simulink model "experimental_1026"  (Simulink 7.5)
settings: Solver=ode1  StartTime=0.0  StopTime=Inf  FixedStep=1/12000  RelTol=1e-3
PostLoadFcn:
  | , if any(exist('dsrtsu_mdlpostloadfcn', 'file') == [2, 3, 6]), try dsrtsu_mdlpostloadfcn('Execute', bdroot); catch fprintf('Error in PostLoadFcn (dsrtsu_mdlpostloadfcn) for model "%s":\n %s\n', bdroot, lasterr); end, end,
InitFcn:
  | iC_ini
values from neighbouring files (symbols this model uses):
  Ts = 0.5    [IMC_calculo_limites_thetas.m]    (also in IMC_datta_ini.m; IMC_ini.m = 8.33333333333e-05; JORGE_controlador_LCL_malha_interna.m = 8.33333333333e-05; LCL_PAPM.m = 8.33333333333e-05)
libraries: powerlib x7, rtilib1103 x2, simulink x1, dsextras x1
CloseFcn:
  | rtwprivate ssgensfun ModelCloseRequest experimental_1021
settings Model: DSRTSU_INTERNAL_RTI_VER=390  DSRTSU_INTERNAL_RTI_TYPE=rti1103  Creator=dpbernardon  LastModifiedBy=dpbernardon  BufferReuse=off
settings SolverCC: InsertRTBMode=Always
settings OptimizationCC: BlockReduction=off  OptimizeBlockIOStorage=off  BufferReuse=off  ExpressionFolding=off  LocalBlockOutputs=off
settings HardwareCC: ProdIntDivRoundTo=Zero  ProdEndianess=BigEndian  ProdHWDeviceType=Generic->Custom  TargetIntDivRoundTo=Zero  TargetEndianess=BigEndian  TargetHWDeviceType=Generic->Custom
settings RTWCC: SystemTargetFile=rti1103.tlc  MakeCommand=make_rti  TemplateMakefile=rti1103.tmf  Description=dSPACE DS1103 Hardware Platform  ProcessScript=rti1103_make_rtw_hook
settings STFCustomTargetCC: ParMdlRefBuildCompliant=on  GeneratePreprocessorConditionals=Disable all  SystemTargetFile=rti1103.tlc
settings GRTTargetCC: CompOptLevelCompliant=off  MatFileLogging=off  ExtModeMexFile=noextcomm
settings CustomProperty: DataType=RTWOptions_EnumType_C__dSPACE RCPHIL 72_matlab_rti1103_tlc_rti1103_1InitialSimState  Value=RUN
settings EnumStrPairs: String=RUN

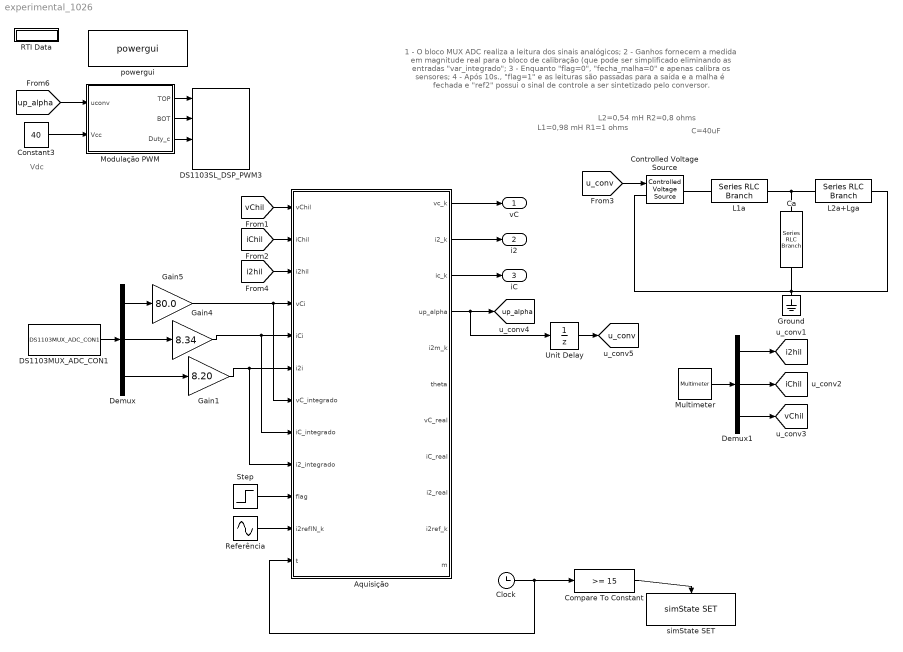
== system experimental_1026 ==
  note: Vdc
  note: 1 - O bloco MUX ADC realiza a leitura dos sinais analógicos;
      | 2 - Ganhos fornecem a medida em magnitude real para o bloco de calibração (que pode ser simplificado  eliminando as entradas "var_integrado";
      | 3 - Enquanto "flag=0", "fecha_malha=0" e apenas calibra os sensores;
      | 4 - Após 10s., "flag=1" e as leituras são passadas para a saída e a malha é fechada e "ref2" possui o sinal de controle a ser sintetizado pelo conversor.
  note: L1=0,98 mH
      | R1=1 ohms
  note: L2=0,54 mH
      | R2=0,8 ohms
  note: C=40uF
  Aquisição : Stateflow chart  TreatAsAtomicUnit=on  SystemSampleTime=Ts
      settings: MinAlgLoopOccurrences=on  RTWSystemCode=Function
  Ca : powerlib/Elements/Series RLC Branch  DialogController=POWERSYS.PowerSysDialog  PhysicalDomain=powersysdomain  SubClassName=unknown  LeftPortType=p1  RightPortType=p1  LConnTagsString=__new0  RConnTagsString=__new0  BranchType=C  Resistance=1  Inductance=1e-3  SetiL0=off  InitialCurrent=0  Capacitance=0.000040  Setx0=off  InitialVoltage=0  Measurements=Branch voltage and current
  Clock : Clock
      settings: Decimation=10
  Compare To Constant : simulink/Logic and Bit Operations/Compare To Constant  SystemSampleTime=-1  relop=>=  const=15  LogicOutDataTypeMode=uint8
  Constant3 : Constant  Value=40  OutDataType=fixdt(1, 16)  OutScaling=2^0
  Controlled Voltage Source : powerlib/Electrical Sources/Controlled Voltage Source  DialogController=POWERSYS.PowerSysDialog  SystemSampleTime=-1  Initialize=on  Source_Type=AC  Amplitude=0  Phase=0  Frequency=0  Measurements=None
  DS1103MUX_ADC_CON1 : rtilib1103/DS1103 MASTER PPC/DS1103MUX_ADC_CON1  SystemSampleTime=-1  ConverterNo=1  ChannelNos=[1 2 3]  TimerAPreTrigger=0  Reserved2=[]  Reserved3=[]  Reserved4=[]  DialogFcn=gui1103mux_adc  UnitName={ 'DS1103MUX_ADC_CON' }  UnitValues={ 1 }  DSProperties=struct('RTI',struct('Version',uint32(1),'BlockType',struct('isSLSource',uint8(1),'isSLSink',uint8(0),'isHWSource',uint8(1),'isHWSink',uint8(0),'isSetup',uint8(0),'isInline',uint8(1),'isNonInline',uint8(0),'isInterrupt',uint8(0),'isChannelwise',uint8(0)),'IOBoardType','DS1103MASTER','UnitType','ADC','Identifier','ADCMUX','DialogType','ML','BlockSet','NONE','SlaveProcessor','NONE'))
  DS1103SL_DSP_PWM3 : rtilib1103/DS1103 SLAVE DSP/DS1103SL_DSP_PWM3  SystemSampleTime=-1  Parameters=[]  TDef=[]  BoardType=[]  PwmMode=[]  Frequency=[]  DeadBand=[]  InitValue=[]  TermMode=[]  TermValue=[]  IntDelay=[]  DialogFcn=[]  Reserved1=[]  Reserved2=[]  Reserved3=[]  Reserved4=[]  Revision=[]  UnitName=[]  UnitValues=[]  DSProperties=struct('RTI',struct('Version',uint32(2),'BlockType',struct('isSLSource',uint8(0),'isSLSink',uint8(1),'isHWSource',uint8(0),'isHWSink',uint8(1),'isSetup',uint8(0),'isInline',uint8(1),'isNonInline',uint8(0),'isInterrupt',uint8(0),'isChannelwise',uint8(0)),'IOBoardType','DS1103SLAVE','UnitType','PWM','Identifier','PWM3','DialogType','ML','BlockSet','NONE','SlaveProcessor','F240'))  RTIBlockInterface=struct('InputPortsActive',[1 1 1 1],'InputPortsWidth',int32([1 1 1 1]),'InputPortsName',{{['Duty cycle a'],['Duty cycle b'],['Duty cycle c'],['PWM Stop']}},'IWork',{{{'',uint32(1)}}},'DialogFcn','rti1103slavepwm3gui','InitLevel',1,'BlockDisplay',{{'','auto'}},'IconTransparency','on','BlockName',struct('Token',{{'DS1103SL_DSP_PWM3'}}))  RTIBlockParameters=struct('PWMFrequency',{{'12000','OFF',[]}},'PWMDeadband',{{'2','OFF',[]}},'PWMPolarityMode',{{[1 1 1 1],'OFF',[]}},'PWMPolarityInvMode',{{[2 2 2 2],'OFF',[]}},'SuspendModeInit',{{[1 1 1],'OFF',[]}},'TTLModeInit',{{[1 1 1],'OFF',[]}},'TTLModeInitNOT',{{[2 2 2],'OFF',[]}},'DutyCycleInitValueCh1',{{'0.5','OFF',[]}},'DutyCycleInitValueCh2',{{'0.5','OFF',[]}},'DutyCycleInitValueCh3',{{'0.5','OFF',[]}},'EnablePWMStop',{{1,'OFF',[]}},'SuspendModeTerm',{{[1 1 1],'OFF',[]}},'TTLModeTerm',{{[1 1 1],'OFF',[]}},'TTLModeTermNOT',{{[2 2 2],'OFF',[]}},'DutyCycleTermValueCh1',{{'0.5','OFF',[]}},'DutyCycleTermValueCh2',{{'0.5','OFF',[]}},'DutyCycleTermValueCh3',{{'0.5','OFF',[]}},'TLCFileName',{{'rti1103pwm3','OFF',[]}})  RTISFcnParameters=struct('PWMFrequency','double','PWMDeadband','double','PWMPolarityMode','double','PWMPolarityInvMode','double','SuspendModeInit','double','TTLModeInit','double','TTLModeInitNOT','double','DutyCycleInitValueCh1','double','DutyCycleInitValueCh2','double','DutyCycleInitValueCh3','double','EnablePWMStop','double','SuspendModeTerm','double','TTLModeTerm','double','TTLModeTermNOT','double','DutyCycleTermValueCh1','double','DutyCycleTermValueCh2','double','DutyCycleTermValueCh3','double','TLCFileName','char')  RTIBlockParaDefault=struct('PWMFrequency',100,'PWMDeadband',50,'PWMPolarityMode',[1 1 1 1],'PWMPolarityInvMode',[2 2 2 2],'SuspendModeInit',[1 1 1],'TTLModeInit',[2 2 2],'TTLModeInitNOT',[1 1 1],'DutyCycleInitValueCh1',0.5,'DutyCycleInitValueCh2',0.5,'DutyCycleInitValueCh3',0.5,'EnablePWMStop',1,'SuspendModeTerm',[1 1 1],'TTLModeTerm',[2 2 2],'TTLModeTermNOT',[1 1 1],'DutyCycleTermValueCh1',0.5,'DutyCycleTermValueCh2',0.5,'DutyCycleTermValueCh3',0.5,'TLCFileName','rti1103pwm3')
  Demux : Demux  Outputs=3
  Demux1 : Demux  Outputs=3
  Gain1 : Gain  Gain=8.20  ParameterDataType=fixdt(1, 16)  ParameterScaling=2^0  OutDataType=fixdt(1, 16)  OutScaling=2^0
  Gain4 : Gain  Gain=8.34  ParameterDataType=fixdt(1, 16)  ParameterScaling=2^0  OutDataType=fixdt(1, 16)  OutScaling=2^0
  Gain5 : Gain  Gain=80.0  ParameterDataType=fixdt(1, 16)  ParameterScaling=2^0  OutDataType=fixdt(1, 16)  OutScaling=2^0
  Ground : powerlib/Elements/Ground  DialogController=POWERSYS.PowerSysDialog  PhysicalDomain=powersysdomain  SubClassName=unknown  LeftPortType=p1  RightPortType=p1  LConnTagsString=a
  L1a : powerlib/Elements/Series RLC Branch  DialogController=POWERSYS.PowerSysDialog  PhysicalDomain=powersysdomain  SubClassName=unknown  LeftPortType=p1  RightPortType=p1  LConnTagsString=__new0  RConnTagsString=__new0  BranchType=RL  Resistance=1  Inductance=0.00098  SetiL0=off  InitialCurrent=0  Capacitance=1e-6  Setx0=off  InitialVoltage=0  Measurements=None
  L2a+Lga : powerlib/Elements/Series RLC Branch  DialogController=POWERSYS.PowerSysDialog  PhysicalDomain=powersysdomain  SubClassName=unknown  LeftPortType=p1  RightPortType=p1  LConnTagsString=__new0  RConnTagsString=__new0  BranchType=RL  Resistance=0.8  Inductance=0.00054  SetiL0=off  InitialCurrent=0  Capacitance=1e-6  Setx0=off  InitialVoltage=0  Measurements=Branch current
  Modulação PWM : Stateflow chart  TreatAsAtomicUnit=on  SystemSampleTime=Ts
      settings: MinAlgLoopOccurrences=on  RTWSystemCode=Function
  Multimeter : powerlib/Measurements/Multimeter  SystemSampleTime=-1  PhasorSimulation=off  OutputType=Complex  sel=[3 2 1]  L=3  Gain=[1 1 1]  yselected={'Ib: L2a+Lga','Ib: Ca','Ub: Ca'};  PSBOutputType=1  PSBequivalent=0  AxesSetting=[0,0.1,-100,100]  Display=0  SavedBlockNames=-11
  RTI Data : Subsystem  Tag=struct('RTIDataServer',struct('RTIDataServerVs','2','RTIModelDescription','struct(''main'',''experimental_1026'',''sub'','''',''isMp'',0)'))  LoadFcn="if exist('rtidc'), try,  rtidc('DataHostBlockClbLoad', gcbh); catch, disp(['Warning: ''LoadFcn'' for RTI Data block failed: ' lasterr]); end, end,"
      settings: CopyFcn="if exist('rtidc'), try,  rtidc('DataHostBlockClbCopy', gcbh); catch, disp(['Warning: ''CopyFcn'' for RTI Data block failed: ' lasterr]); end, end,"  DeleteFcn="if exist('rtidc'), try,  rtidc('DataHostBlockClbDelete', gcbh); catch, disp(['Warning: ''DeleteFcn'' for RTI Data block failed: ' lasterr]); end, end,"  ModelCloseFcn="if exist('rtidc'), try,  rtidc('DataHostBlockClbModelClose', gcbh); catch, disp(['Warning: ''ModelCloseFcn'' for RTI Data block failed: ' lasterr]); end, end,"  PreSaveFcn="if exist('rtidc'), try,  rtidc('DataHostBlockClbPreSave', gcbh); catch, disp(['Warning: ''PreSaveFcn'' for RTI Data block failed: ' lasterr]); end, end,"  PostSaveFcn="if exist('rtidc'), try,  rtidc('DataHostBlockClbPostSave', gcbh); catch, disp(['Warning: ''PostSaveFcn'' for RTI Data block failed: ' lasterr]); end, end,"  NameChangeFcn="if exist('rtidc'), try,  rtidc('DataHostBlockClbNameChange', gcbh); catch, disp(['Warning: ''NameChangeFcn'' for RTI Data block failed: ' lasterr]); end, end,"
      mask Type: RTI_DATA_HOST
      mask Description:
      | RTI Data Block.
      | This block is used by RTI to store internal model-dependent data.
      | Please keep this block on the root level of the model. Deleting this block will result in data loss.
      | 
      | NEVER DELETE OR COPY THIS BLOCK!
      mask Help:
      | RTI Data Block.
      | This block is used by RTI to store internal model-dependent data.
      | Please keep this block on the root level of the model. Deleting this block will result in data loss.
      | 
      | NEVER DELETE OR COPY THIS BLOCK!
      mask Display:
      | text(0.5, 0.5, 'RTI Data', 'HorizontalAlignment', 'center');
      | plot([1 0]);
  Referência : Sin  Amplitude=5  Bias=0  Frequency=2*pi*60  Phase=0  Samples=10  SampleTime=1/12000  Offset=0
  Step : Step  Time=10  SampleTime=0
  Unit Delay : UnitDelay  SampleTime=-1
  powergui : powerlib/powergui  Priority=1  SystemSampleTime=-1  SimulationMode=Discrete  SampleTime=Ts  frequency=60  SPID=off  DisableSnubberDevices=off  DisableRonSwitches=off  DisableVfSwitches=off  SwTol=0  Interpol=off  frequencyindice=0  echomessages=off  HookPort=off  DisplayEquations=off  FunctionMessages=off  EnableUseOfTLC=off  x0status=blocks  RestoreLinks=warning  ResistiveCurrentMeasurement=off  Frange=[0:2:500]  Ylog=off  Xlog=on  ShowGrid=off  save=off  variable=ZData  ZoomFFT=off  StartTime=0.0  cycles=1  DisplayStyle=1  fundamental=60  FreqAxis=off  MaxFrequency=1000  frequencyindicesteady=1  RmsSteady=1  display=off  Ts=0  methode=off
  simState SET : dsextras/simState SET  SystemSampleTime=-1  TriggerPort=rising  EnablePort=none  SimStateMode=PAUSE  TLCFileName=rti_simstate_set  Reserved1=[]  Reserved2=[]  Reserved3=[]  Reserved4=[]  DSProperties=struct('RTI',struct('Version',uint32(1),'BlockType',struct('isSLSource',uint8(1),'isSLSink',uint8(0),'isHWSource',uint8(0),'isHWSink',uint8(0),'isSetup',uint8(0),'isInline',uint8(1),'isNonInline',uint8(0),'isInterrupt',uint8(0),'isChannelwise',uint8(0)),'IOBoardType','EXTRAS','UnitType','SIMSTATESET','Identifier','SIMSTATESET','DialogType','SL','BlockSet','NONE','SlaveProcessor','NONE'))  RTIBlockInterface=struct('OutputPortsWidth',int32(0),'BlockDisplay',{{['simState PAUSE'],'center'}},'IconTransparency','on','InitLevel',2,'BlockName',struct('Token',{{['simState SET']}}),'TriggerPort',{{'rising'}},'EnablePort',{{'none'}},'MaskDescription',['Set simState to the specified value when the block is executed.'])  RTIBlockParameters=struct('TriggerPort',{{2,'OFF',[]}},'EnablePort',{{1,'OFF',[]}},'SimStateMode',{{2,'OFF',[]}},'TLCFileName',{{'rti_simstate_set','OFF',[]}})  RTISFcnParameters=struct('TriggerPort','double','EnablePort','double','SimStateMode','char','TLCFileName','char')  RTIBlockParaDefault=struct('TriggerPort',2,'EnablePort',1,'SimStateMode',1,'TLCFileName','rti_simstate_set')
  vC : Outport  OutDataType=fixdt(1, 16)  OutScaling=2^0
  i2 : Outport  Port=2  OutDataType=fixdt(1, 16)  OutScaling=2^0
  iC : Outport  Port=3  OutDataType=fixdt(1, 16)  OutScaling=2^0
  tag scope: i2hil=global, iChil=global, u_conv=global, up_alpha=global, vChil=global
  wires:
  DS1103MUX_ADC_CON1/1 -> Demux/1
  Step/1 -> Aquisição/10(flag)
  Demux/2 -> Gain4/1
  Demux/3 -> Gain1/1
  Aquisição/3(ic_k) -> iC/1
  Demux/1 -> Gain5/1
  Aquisição/1(vc_k) -> vC/1
  Aquisição/2(i2_k) -> i2/1
  Multimeter/1 -> Demux1/1
  Demux1/1 -> [i2hil]
  Demux1/2 -> [iChil]
  Modulação PWM/1(TOP) -> DS1103SL_DSP_PWM3/1
  Modulação PWM/2(BOT) -> DS1103SL_DSP_PWM3/2
  Modulação PWM/3(Duty_c) -> DS1103SL_DSP_PWM3/3
  Constant3/1 -> Modulação PWM/2(Vcc)
  Compare To Constant/1 -> simState SET/Trigger
  Aquisição/4(up_alpha) -> [up_alpha], Unit Delay/1
  Demux1/3 -> [vChil]
  [vChil] -> Aquisição/1(vChil)
  [i2hil] -> Aquisição/3(i2hil)
  [iChil] -> Aquisição/2(iChil)
  Gain5/1 -> Aquisição/4(vCi), Aquisição/7(vC_integrado)
  Gain1/1 -> Aquisição/6(i2i), Aquisição/9(i2_integrado)
  Gain4/1 -> Aquisição/5(iCi), Aquisição/8(iC_integrado)
  [up_alpha] -> Modulação PWM/1(uconv)
  Unit Delay/1 -> [u_conv]
  [u_conv] -> Controlled Voltage Source/1
  Clock/1 -> Compare To Constant/1, Aquisição/12(t)
  Referência/1 -> Aquisição/11(i2refIN_k)
  connections:
  L2a+Lga/LConn1 -- L1a/RConn1 -- Ca/LConn1
  Controlled Voltage Source/RConn1 -- L1a/LConn1
  L2a+Lga/RConn1 -- Ca/RConn1 -- Controlled Voltage Source/LConn1 -- Ground/LConn1

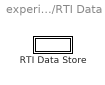
== system experimental_1026/RTI Data ==
  RTI Data Store : Subsystem  Tag="struct('private',struct('version',struct('dsVer',uint32(2),'dsVerCreation',uint32(2),'RTI',struct('ver','6.8','type','RTI1103')),'access',struct('type','Model','isPerm',1,'created',['15-Dec-2012 18:39:02'],'modified',['31-Oct-2013 17:53:13'],'location','')),'public',struct('main',struct('data',[]),'sub',struct('name',{{'experimental_1026'}},'data',{{struct('TH',struct('thTaskInfo',struct('taskType',{'TIMER','HWINT','TMRINT','SWINT'},'tasksNumOf',{1,0,0,0},'srcIds',{{'TIMERA'},{},{},{}},'taskNames',{{['Timer Task 1']},{},{},{}})),'th_tc',struct('dataType','TASK','taskGroupId','','taskGroupList',{{}},'taskSchedulingPolicy','FCFS','taskType','TIMER','blkh',-1,'srcId','TIMERA','srcSgnName',['Timer A interrupt'],'srcCpuName','','taskName',['Timer Task 1  [8.33333e-005] s'],'taskNameDisplayExt','','smplTime',8.3333333333333331e-05,'smplTimeOffs',0,'hasFixedPriority',0,'priority',1,'hasFixedOvc',0,'ovcType',1,'ovcMax',1),'tc_th',struct('dataType','TASK','taskGroupId','','taskGroupList',{{}},'taskSchedulingPolicy','FCFS','taskType','TIMER','blkh',-1,'srcId','TIMERA','srcSgnName',['Timer A interrupt'],'srcCpuName','','taskName',['Timer Task 1  [8.33333e-005] s'],'taskNameDisplayExt','','smplTime',8.3333333333333331e-05,'smplTimeOffs',0,'hasFixedPriority',0,'priority',1,'hasFixedOvc',0,'ovcType',1,'ovcMax',1))}})))"
      mask Type: RTI_DATA_STORE
      mask Description:
      | RTI Data Store Block. This block is used by RTI to store internal model dependent data. Deleting this block will result in data loss.
      | 
      | NEVER DELETE, COPY, OR MODIFY THIS BLOCK!
      mask Help:
      | RTI Data Store Block. This block is used by RTI to store internal model dependent data. Deleting this block will result in data loss.
      | 
      | NEVER DELETE, COPY, OR MODIFY THIS BLOCK!
      mask Display: text(0.5, 0.5, ' ', 'HorizontalAlignment', 'center');

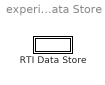
== system experimental_1026/RTI Data/RTI Data Store ==
  RTI Data Store : Subsystem
      mask Type: RTI_DATA_STORE
      mask Description:
      | RTI Data Store Block. This block is used by RTI to store internal model dependent data. Deleting this block will result in data loss.
      | 
      | NEVER DELETE, COPY, OR MODIFY THIS BLOCK!
      mask Help:
      | RTI Data Store Block. This block is used by RTI to store internal model dependent data. Deleting this block will result in data loss.
      | 
      | NEVER DELETE, COPY, OR MODIFY THIS BLOCK!
      mask Display: text(0.5, 0.5, ' ', 'HorizontalAlignment', 'center');

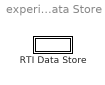
== system experimental_1026/RTI Data/RTI Data Store/RTI Data Store ==
  RTI Data Store : Subsystem
      mask Type: RTI_DATA_STORE
      mask Description:
      | RTI Data Store Block. This block is used by RTI to store internal model dependent data. Deleting this block will result in data loss.
      | 
      | NEVER DELETE, COPY, OR MODIFY THIS BLOCK!
      mask Help:
      | RTI Data Store Block. This block is used by RTI to store internal model dependent data. Deleting this block will result in data loss.
      | 
      | NEVER DELETE, COPY, OR MODIFY THIS BLOCK!
      mask Display: text(0.5, 0.5, ' ', 'HorizontalAlignment', 'center');

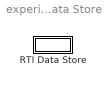
== system experimental_1026/RTI Data/RTI Data Store/RTI Data Store/RTI Data Store ==
  RTI Data Store : Subsystem
      mask Type: RTI_DATA_STORE
      mask Description:
      | RTI Data Store Block. This block is used by RTI to store internal model dependent data. Deleting this block will result in data loss.
      | 
      | NEVER DELETE, COPY, OR MODIFY THIS BLOCK!
      mask Help:
      | RTI Data Store Block. This block is used by RTI to store internal model dependent data. Deleting this block will result in data loss.
      | 
      | NEVER DELETE, COPY, OR MODIFY THIS BLOCK!
      mask Display: text(0.5, 0.5, ' ', 'HorizontalAlignment', 'center');

== system experimental_1026/RTI Data/RTI Data Store/RTI Data Store/RTI Data Store/RTI Data Store ==

== matlab function Aquisição ==
  data: vChil input double; iChil input double; i2hil input double; vCi input double; vc_k output double; iCi input double; i2i input double; vC_integrado input double; iC_integrado input double; i2_integrado input double; flag input double; i2_k output double; ic_k output double; up_alpha output double; i2m_k output double; theta output double; vC_real output double; iC_real output double; i2_real output double; i2ref_k output double; i2refIN_k input double; m output double; t input double
function [vc_k,i2_k,ic_k,up_alpha,i2m_k,theta,vC_real,iC_real,i2_real,i2ref_k,m] = Controle(vChil, iChil, i2hil, vCi,iCi,i2i,vC_integrado,iC_integrado,i2_integrado,flag,i2refIN_k,t)
%#CODEGEN

%%%%%%%%%%%%%%%%%%%%%%%%%%%%%%%%%%%%%%%%%%%%%%%%%%%%%%%%%%%%%%%%%%%%%%%%%%%
% Inicializações do controlador

%%Kp=k*Ts/(L1+L2)
%Kp=0.3;
Kp=0.183;
%Kp=0.1487;
%kp=5.23;
kp=3.35;
%kp=1.91;

%polos do modelo de referência:
p1=0.5; %0.3
p2=0.5;

km=(1-p1)*(1-p2);

%constantes -> gamaD < (1-gama)*km/kp
gamaD=0.01; %0.1
gama=0.95; %0.95

delta0=0.98; %0.97

hil=0;

%% Variáveis Persistentes do Controlador
persistent theta_k;
if isempty(theta_k)
    %theta_k=[-0.03; -0.36; -0.57; -0.01; 0.16; 0.02];
    %theta_k=[-0.6; 0; -2.2; 2.2; 0; 0]; % Calculado para os novos núcleos de ar
    %theta_k=[-0.6; 0; -3.5; 3.5; 0; 0]; %L1=1m L2=0.5m e C=80u; kp=5.23 Kp=0.3
    %theta_k=[-1.2; 3.14; -3.3; 2.23; 0; 0];
    %theta_k=[-1.2; -1.63; -1.85; 3.48; 0; 0];
    %theta_k=[-0.8; 1.08; -1.6; 2.67; 0; 0];
    theta_k=[0; 0; -1.36; 1.36; 0; 0];
    %theta_k=[0.24; 0.16; -1.2; 1.62; 0; 0]; %realimentados da medida experimental
    %theta_k=[-0.6; 0; -10; 10; 0; 0];
    %theta_k=[-0.6; 0; -4.3; 4.3; 0; 0]; %parametros para L1=L2=0.5m e C=80u
end

persistent omega_k;
if isempty(omega_k)
    omega_k=[0; 0; 0; 0; 0; 0];
end

persistent omega_k_1;
if isempty(omega_k_1)
    omega_k_1=[0; 0; 0; 0; 0; 0];
end

persistent omega_k_2;
if isempty(omega_k_2)
    omega_k_2=[0; 0; 0; 0; 0; 0];
end

persistent eta_k_1;
if isempty(eta_k_1)
    eta_k_1=[0; 0; 0; 0; 0; 0];
end

persistent eta_k_2;
if isempty(eta_k_2)
    eta_k_2=[0; 0; 0; 0; 0; 0];
end

persistent i2m_k_1;
if isempty(i2m_k_1)
    i2m_k_1=0;
end

persistent i2m_k_2;
if isempty(i2m_k_2)
    i2m_k_2=0;
end

persistent i2ref_k_1;
if isempty(i2ref_k_1)
    i2ref_k_1=0;
end

persistent i2ref_k_2;
if isempty(i2ref_k_2)
    i2ref_k_2=0;
end

persistent v_k_1;
if isempty(v_k_1)
    v_k_1=0;
end

persistent v_k_2;
if isempty(v_k_2)
    v_k_2=0;
end

persistent rho_k;
if isempty(rho_k)
    rho_k=Kp/km;
end

persistent m2;
if isempty(m2)
    m2=1;
end

persistent u_k_1;
if isempty(u_k_1)
    u_k_1=0;
end

persistent u_k_2;
if isempty(u_k_2)
    u_k_2=0;
end

persistent timer;
if isempty(timer)
    timer=0;
end


%% Variáveis Persistentes para Calibração
persistent vC_avg;
if isempty(vC_avg)
    vC_avg=0;
end

persistent i2_avg;
if isempty(i2_avg)
    i2_avg=0;
end

persistent iC_avg;
if isempty(iC_avg)
    iC_avg=0;
end

persistent flag1;
if isempty(flag1)
    flag1=0;
end

%%%%%%%%%%%%%%%%%%%%%%%%%%%%%%%%%%%%%%%%%%%%%%%%%%%%%%%%%%%%%%%%%%%%%%%%%%%
%% Algoritmo de calibração
if flag<1
    flag1=0;
end

if flag<1
    vC_avg = vC_avg + vC_integrado*1/12000;
    i2_avg = i2_avg + i2_integrado*1/12000;
    iC_avg = iC_avg + iC_integrado*1/12000;
elseif flag1==0
    flag1=1;
    vC_avg = vC_avg/10;
    i2_avg = i2_avg/10;
    iC_avg = iC_avg/10;
end

% Disponibiliza as aquisições na saída
if flag1>0
    
    if hil>0
        vc_k = vChil;
        ic_k = iChil;
        i2_k = i2hil;
    else
        vc_k= vCi - vC_avg;
        ic_k= iCi - iC_avg;
        i2_k= i2i - i2_avg;        
    end
    
    vC_real= vCi - vC_avg;
    iC_real= iCi - iC_avg;
    i2_real= i2i - i2_avg;
    
    %%%%%%%%%%%%%%%%%%%%%%%%%%%%%%%%%%%%%%%%%%%%%%%%%%%%%%%%%%%%%%%%%%%%%%%
    % Controle
    %%%%%%%%%%%%%%%%%%%%%%%%%%%%%%%%%%%%%%%%%%%%%%%%%%%%%%%%%%%%%%%%%%%%%%%
    %Ação de controle
    if timer<1
        i2ref_k= i2refIN_k*timer;
        timer=timer+0.001; % 5 ciclos de 60Hz (200 samples)
    else
        i2ref_k=i2refIN_k;
    end
    
    if t>11
        i2ref_k = -i2refIN_k;
    end
    
    omega_k(3)= i2_k;
    omega_k(4)= i2ref_k;
    omega_k(5)= 0;
    omega_k(6)= 0;

    u_k= theta_k'*omega_k;

    % Controlador P
    up_alpha= kp*(u_k-ic_k);
    %up_alpha=u_k;

    eta_k= (p1+p2)*eta_k_1 - p1*p2*eta_k_2 + (1-p1)*(1-p2)*omega_k_2;

    i2m_k= (p1+p2)*i2m_k_1 - p1*p2*i2m_k_2 + (1-p1)*(1-p2)*i2ref_k_2;

    e1_k= i2_k - i2m_k;

    v_k= (p1+p2)*v_k_1 - p1*p2*v_k_2 + (1-p1)*(1-p2)*u_k_2;

    q_k= theta_k'*eta_k;

    e2_k= -v_k+q_k;

    ea_k= e1_k+rho_k*e2_k;

    m2_k= eta_k'*eta_k + e2_k^2 + m2;
    m=m2_k;


    %% Atualização

    ea_m2=ea_k/m2_k;

    %calcula theta(k+1)
    theta_k = theta_k - (gamaD*ea_m2)*eta_k;
    theta = theta_k;

    %calcula rho(k+1)
    rho_k= rho_k - gama*e2_k*ea_m2;

    m2 = delta0*(m2 - 1) + u_k*u_k + i2_k*i2_k + 1;

    omega_k_2=omega_k_1;
    omega_k_1=omega_k;

    omega_k(1)=0.05*omega_k(1) + 1*u_k; %0.5 e 0.5
    omega_k(2)=0.05*omega_k(2) + 1*i2_k;

    eta_k_2=eta_k_1;
    eta_k_1=eta_k;

    i2ref_k_2 = i2ref_k_1;
    i2ref_k_1 = i2ref_k;

    i2m_k_2=i2m_k_1;
    i2m_k_1=i2m_k;

    v_k_2=v_k_1;
    v_k_1=v_k;

    u_k_2=u_k_1;
    u_k_1=u_k;
    %%%%%%%%%%%%%%%%%%%%%%%%%%%%%%%%%%%%%%%%%%%%%%%%%%%%%%%%%%%%%%%%%%%%%%%
else
    vC_real = vCi - vC_avg;
    i2_real = i2i - i2_avg;
    iC_real = iCi - iC_avg;
    
    vc_k = vChil;
    ic_k = iChil;
    i2_k = i2hil;
    
    m=0;
    i2ref_k=0;
    i2m_k=0;
    theta=theta_k;
    up_alpha=0;
end


end

== matlab function Modulação PWM ==
  data: uconv input double; TOP output double; BOT output double; Vcc input double; Duty_c output double
function [TOP,BOT,Duty_c] = modulacao(uconv,Vcc)

%#CODEGEN
u=-uconv/Vcc;
TOP=0;
BOT=0;

if u>0
    TOP=u;
    BOT=0;
end

if u<0
    TOP=0;
    BOT=-u;
end

Duty_c=0;

end
